simulink model "Tx_OFDM"  (R2023a)
settings: Solver=FixedStepAuto  StartTime=0.0  StopTime=10.0  RelTol=1e-3
model workspace (MAT data in the model file):
  bit_per_symbol = 2
  fsc = 10000
  fsp = 150000
  stime = 0.0001
  symbol = 1
libraries: hdlsllib x4, commrandsrc2 x1, dsphdlxfrm2 x1, whdlmod x1, commdigbbndpm3 x1
settings Model: Creator=acer  LastModifiedBy=acer
settings OptimizationCC: BlockReduction=off  ConditionallyExecuteInputs=off  EnhancedBackFolding=on  PassReuseOutputArgsAs=Individual arguments  ZeroExternalMemoryAtStartup=off  ZeroInternalMemoryAtStartup=off  MaxStackSize=64  OptimizeBlockOrder=speed  DifferentSizesBufferReuse=on  OptimizationCustomize=off  EfficientTunableParamExpr=on
settings DebuggingCC: ParameterTunabilityLossMsg=error
settings HardwareCC: ProdBitPerPointer=32  ProdBitPerSizeT=32  ProdBitPerPtrDiffT=32  ProdLargestAtomicInteger=Long  ProdLargestAtomicFloat=Double  ProdWordSize=32  ProdHWDeviceType=ARM Compatible->ARM Cortex
settings SFSimCC: MATLABDynamicMemAlloc=off
settings RTWCC: Description=Embedded Coder  SystemTargetFile=ert.tlc  TLCOptions="-aInlineSetEventsForThisBaseRateFcn=TLC_FALSE -aSuppressMultiTaskScheduler=TLC_FALSE  -aRateBasedStepFcn=0"  TemplateMakefile=ert_default_tmf
settings CodeAppCC: ForceParamTrailComments=on  IgnoreCustomStorageClasses=off  OperatorAnnotations=on  SimulinkDataObjDesc=on  SFDataObjDesc=on  InsertBlockDesc=on

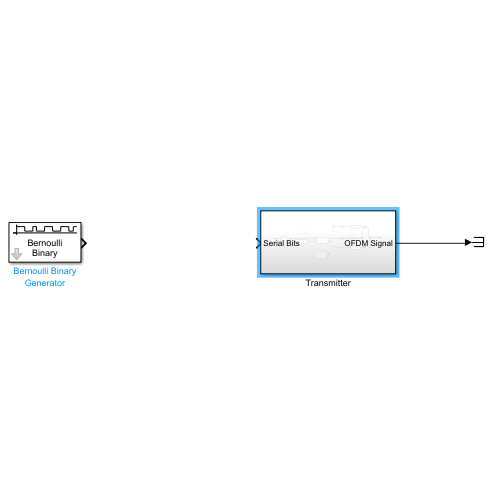
[thumbnail: Simulink's stored preview of the top-level diagram]
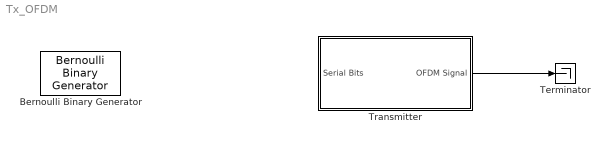
== system Tx_OFDM ==
  Bernoulli Binary Generator : commrandsrc2/Bernoulli Binary Generator  P=0.5  seed=61  Ts=stime  frameBased=on  sampPerFrame=symbol * bit_per_symbol  orient=off  outDataType=boolean
  Terminator : Terminator
  Transmitter : Subsystem
  wires:
  Transmitter/1(OFDM Signal) -> Terminator/1

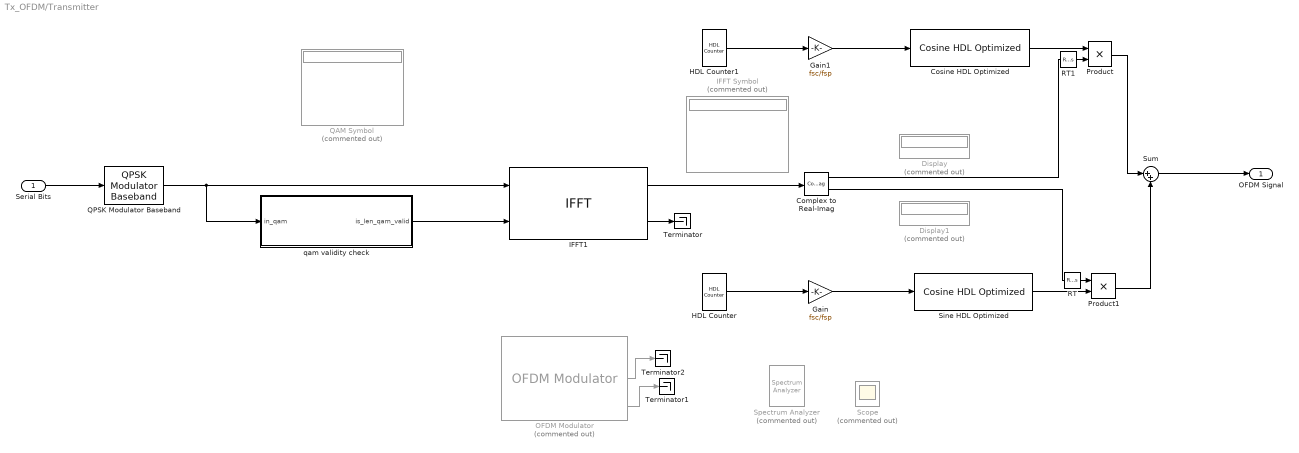
== system Tx_OFDM/Transmitter ==
  Serial Bits : Inport  OutDataTypeStr=int8
  Complex to Real-Imag : ComplexToRealImag
  Cosine HDL Optimized : hdlsllib/Lookup Tables/Cosine HDL Optimized  OutputFormula=cos(2*pi*u)  NumDataPoints=64  TableDataTypeStr=fixdt(0,16,15)  SimulateLUTROMDelay=off
  Display : Display  Commented=on
  Display1 : Display  Commented=on
  Gain : Gain  Gain=fsc/fsp
  Gain1 : Gain  Gain=fsc/fsp
  HDL Counter : hdlsllib/Sources/HDL Counter  CountType=Modulo  CountInit=0  CountStep=1  CountMax=fsp  CountFromType=Specify  CountFrom=0  CountResetPort=off  CountLoadPort=off  CountEnbPort=off  CountDirPort=off  CountHitOutputPort=off  CountDataType=Signed  CountWordLen=32  CountFracLen=0  CountSampTime=1/fsp
  HDL Counter1 : hdlsllib/Sources/HDL Counter  CountType=Modulo  CountInit=0  CountStep=1  CountMax=fsp  CountFromType=Specify  CountFrom=0  CountResetPort=off  CountLoadPort=off  CountEnbPort=off  CountDirPort=off  CountHitOutputPort=off  CountDataType=Signed  CountWordLen=32  CountFracLen=0  CountSampTime=1/fsp
  IFFT Symbol : Display  Commented=on
  IFFT1 : dsphdlxfrm2/IFFT  FFTLength=64  Architecture=Streaming Radix 2^2  ComplexMultiplication=Use 4 multipliers and 2 adders  BitReversedOutput=on  BitReversedInput=off  Normalize=on  SimulateUsing=Code generation  RoundingMethod=Floor  ResetInputPort=off  StartOutputPort=off  EndOutputPort=off
  OFDM Modulator : whdlmod/OFDM Modulator  Commented=on  OFDMParametersSource=Property  FFTLength=64  MaxFFTLength=64  CPLength=0  numLgSc=0  numRgSc=0  InsertDCNull=off  Windowing=off  WindowLength=4  MaxWindowLength=8  ResetInputPort=off  Normalize=on  RoundingMethod=Floor  SimulateUsing=Code generation
  Product : Product
  Product1 : Product  OutDataTypeStr=fixdt(1,16,0)
  QAM Symbol : Display  Commented=on
  QPSK Modulator Baseband : commdigbbndpm3/QPSK Modulator Baseband  InType=Integer  Enc=Gray  Ph=pi/4  outDtype=Fixed-point  outWordLen=16  outUDDataType=sfix(16)  outFracLenMode=Best precision  outFracLen=15  outDataTypeStr=fixdt(1,16)  outLastDataTypeStr=fixdt(1,16)
      settings: LibrarySourceBlock=|
      | commhdldigbbndpm/QPSK
      | Modulator
      | Baseband
  RT : RateTransition  OutPortSampleTime=6.666666666666667e-06
  RT1 : RateTransition  OutPortSampleTime=6.666666666666667e-06
  Scope : Scope  Commented=on
  Sine HDL Optimized : hdlsllib/Lookup Tables/Cosine HDL Optimized  OutputFormula=sin(2*pi*u)  NumDataPoints=64  TableDataTypeStr=fixdt(0,16,15)  SimulateLUTROMDelay=off
      settings: LibrarySourceBlock=|
      | hdlsllib/Lookup
      | Tables/Sine
      | HDL Optimized
  Spectrum Analyzer : SpectrumAnalyzer  Commented=on  WindowPosition=[699.000000,188.000000,800.000000,489.000000,]  ScopeFrameLocation=window  Span=9600000  StartFrequency=-4800000  StopFrequency=4800000  SpectrumUnits=dBW  YLimits=[-86.59648917,2.84755915]  ColorLimits=[-20 80]  ShowLegend=on  DefaultConfigurationName=spbscopes.SpectrumAnalyzerBlockCfg  IsFrequencyInputMode=0  FrequencyVectorPort=0  FrequencyVectorFromPort=0  FrequencyInputRBWPort=0  FrequencyInputRBWFromPort=0
  Sum : Sum  Inputs=|++
  Terminator : Terminator
  Terminator1 : Terminator
  Terminator2 : Terminator
  qam validity check : MATLAB Function  TreatAsAtomicUnit=on
  OFDM Signal : Outport
  wires:
  Serial Bits/1 -> QPSK Modulator Baseband/1
  IFFT1/2 -> Terminator/1
  Gain1/1 -> Cosine HDL Optimized/1
  Gain/1 -> Sine HDL Optimized/1
  Cosine HDL Optimized/1 -> Product/1
  Sine HDL Optimized/1 -> Product1/2
  Complex to Real-Imag/1 -> RT1/1
  Complex to Real-Imag/2 -> RT/1
  Product/1 -> Sum/1
  Product1/1 -> Sum/2
  Sum/1 -> OFDM Signal/1
  OFDM Modulator/3 -> Terminator1/1
  OFDM Modulator/2 -> Terminator2/1
  qam validity check/1(is_len_qam_valid) -> IFFT1/2
  QPSK Modulator Baseband/1 -> IFFT1/1, qam validity check/1(in_qam)
  IFFT1/1 -> Complex to Real-Imag/1
  HDL Counter/1 -> Gain/1
  HDL Counter1/1 -> Gain1/1
  RT/1 -> Product1/1
  RT1/1 -> Product/2

== matlab function Tx_OFDM/Transmitter/qam validity check ==
  data: in_qam input; is_len_qam_valid output
function is_len_qam_valid = fcn(in_qam)
%#codegen
max_prime_factor = max(factor(length(in_qam)));

if(max_prime_factor == 2)
    is_len_qam_valid = true;
else 
    is_len_qam_valid = false;
end
